simulink model "MotorImplementation"  (R2022a)
settings: Solver=FixedStepAuto  StartTime=0.0  StopTime=60  FixedStep=1/25  RelTol=1e-3
model workspace (MATLAB code in the model file):
  | %% Mechanical Parameters
  | d_Drum = 23.23e-2; % Meter
  | Drum_Friction = 0.001; % Ns/m
  | Drum_Inertia = 1.0; %kgm^2
  | 
  | n_sh = 5;
  | 
  | %% Load Case 1
  | Hs = 2.2; % m
  | T_w = 8.0; % s
  | m_payload = 8000; % kg
  | h_payload_0 = 75; % m
  | h_payload_final = h_payload_0; % m
  | h_seabed = 350; % m
  | 
  | %% Load Case 2
  | Hs = 2.2; % m
  | T_w = 8.0; % s
  | m_payload = 8000; % kg
  | h_payload_0 = 75; % m
  | h_payload_final = 15; % m
  | h_seabed = 350; % m
  | 
  | %% Load Case 3
  | Hs = 2.2; % m
  | T_w = 8.0; % s
  | m_payload = 8000; % kg
  | h_payload_0 =15; % m
  | h_payload_final = 0; % m
  | h_seabed = 350; % m
  | 
  | %% Sensors
  | % Noise simulation
  | sigma_w = 0.5; %m/s^2 (Standard deviation of noise)
  | beta = 10000; % Positive constant [-]
  | 
  | %% Payload parameters
  | % mass already defined (8000kg)
  | Volume_pl = 2; %m^3
  | Area_pl = 1.5; %m^2
  | C_D = 1.8; %[-] Drag coefficient
  | 
  | %syms rho vel
  | %F_drag = 0.5 * rho * vel^2 * C_D * Area_pl; % Density of sea water(surface) approx 1.025 kg/m^3, velocity comes from the simulation.
  | 
  | %% Seabed
  | k_spring = 1.8e6; %N/m
  | b_damper = 6.5e5; %Ns/m
  | rho = 1.025;
  | %syms delta_x
  | %if delta_x < 0
  | %    F_sb = 0;
  | %else
  | %    F_sb = k_spring*delta_x + b_damper*vel*sqrt(delta_x);
  | %end
  | 
  | %% Bouyant force
  | % The force pushing upwards when something floats down in water. Dependend
  | % on the fluid density, volume of the object falling and gravity
  | g = 9.81;
  | %F_boy = rho * Volume_pl * g;
  | 
  | %% Mechanical Parameters
  | T_N = 579 % Nominal torque [Nm]
  | PF_N = 0.85; % Nominal power factor
  | f=50;
  | n_N = 1483; % mechanical speed [rpm]
  | P_N = 90000 % Nominal mechanical power [W]
  | U = 400; % line-to-line rms stator voltage [V]
  | eta_N = 0.947; % efficiency
  | n_p = 2; % pole pairs
  | I_N=160;
  | 
  | %% Electrical parameters
  | % T-circuit
  | Rs = 0.04264;
  | L_sl = 0.3172;
  | Lm = 5.3031;
  | L_rl = 0.3172;
  | R_R = 0.0288;
  | psi_R = 20*P_N/(sqrt(2)*pi*n_p*I_N*n_N);
  | %Inv Gamma Transform
  | Lr = 5.3031 + 0.3172;
  | L_M = 5.3031^2/Lr;
  | L_M_hat = 5;
  | 
  | PSI_R = 5.3031/Lr * psi_R;
  | L_sigma =((5.3031+0.3172) - Lr);
  | %L_sigma_hat = 0.12;
  | RR = (5.3031/Lr)^2 * 0.0288;
  | %RR_Hat = 0.025;
  | R_R_opt = 0.0193;
  | X_M_opt = 2.81;
  | X_sig_opt = 0.0445;
  | 
  | R_R_hat = 0.02;
  | X_M_hat = 3;
  | X_sig_hat = 0.05;
  | R_s = 0.04264;
  | %% Control parameters
  | omega_bw = log(9)/1e-3;
  | kp = omega_bw * X_sig_hat;
  | ki = omega_bw^2 * X_sig_hat;
undefined symbols (not defined in the file): I_max, L_sigma_hat, magnitude, omega_1_N, psi_ref, R_hat, RR_Hat, Ts, V_base, w_BW
libraries: fl_lib x22, nesl_utility x10, CustomComponents_lib x6, slpidlib x4, simulink x3, eeTransforms x2, sdl_lib x1
(part 2 of 2)

== system MotorImplementation/Field Oriented Control/Velocity Controller ==
  omega_ref : Inport
  omega_rotor : Inport  Port=2
  PID Controller : slpidlib/PID Controller  Controller=PID  Form=Parallel  TimeDomain=Discrete-time  UseExternalTs=off  SampleTime=-1  IntegratorMethod=Forward Euler  FilterMethod=Forward Euler  ControllerParametersSource=internal  P=100  I=1000  UseKiTs=off  D=0  N=100  UseFilter=on  TunerSelectOption=Transfer Function Based (PID Tuner App)  InitialConditionSource=internal  InitialConditionForIntegrator=0  InitialConditionForFilter=0  DifferentiatorICPrevScaledInput=0  ExternalReset=none  TrackingMode=off  Kt=1  LimitOutput=off  SatLimitsSource=internal  UpperSaturationLimit=inf  LowerSaturationLimit=-inf  LinearizeAsGain=on  AntiWindupMode=none  Kb=1  POutMin=[]  POutMax=[]  IOutMin=[]  IOutMax=[]  DOutMin=[]  DOutMax=[]  NOutMin=[]  NOutMax=[]  SumOutMin=[]  SumOutMax=[]  SaturationOutMin=[]  SaturationOutMax=[]  PParamMin=[]  PParamMax=[]  IParamMin=[]  IParamMax=[]  DParamMin=[]  DParamMax=[]  NParamMin=[]  NParamMax=[]  KbParamMin=[]  KbParamMax=[]  KtParamMin=[]  KtParamMax=[]  KbOutMin=[]  KbOutMax=[]  KtOutMin=[]  KtOutMax=[]  IntegratorOutMin=[]  IntegratorOutMax=[]  FilterOutMin=[]  FilterOutMax=[]  SumI1OutMin=[]  SumI1OutMax=[]  SumI2OutMin=[]  SumI2OutMax=[]  SumI3OutMin=[]  SumI3OutMax=[]  SumI4OutMin=[]  SumI4OutMax=[]  SumDOutMin=[]  SumDOutMax=[]  DifferentiatorOutMin=[]  DifferentiatorOutMax=[]  FilterDiffOutCoefMin=[]  FilterDiffOutCoefMax=[]  ReciprocalOutMin=[]  ReciprocalOutMax=[]  SumDenOutMin=[]  SumDenOutMax=[]  SumNumOutMin=[]  SumNumOutMax=[]  DivideOutMin=[]  DivideOutMax=[]  UdiffTsProdOutMin=[]  UdiffTsProdOutMax=[]  NTsProdOutMin=[]  NTsProdOutMax=[]  UintegralTsProdOutMin=[]  UintegralTsProdOutMax=[]  UngainTsProdOutMin=[]  UngainTsProdOutMax=[]  IntegratorContinuousStateAttributes=''  IntegratorStateMustResolveToSignalObject=off  IntegratorRTWStateStorageClass=Auto  FilterContinuousStateAttributes=''  FilterStateMustResolveToSignalObject=off  FilterRTWStateStorageClass=Auto  ParallelPVariant=InternalParameters  IdealPVariant=Disabled  IVariant=InternalParameters  DVariant=InternalParameters  IntegratorVariant=Discrete  SatVariant=Disabled  AWVariant=Passthrough  PCopyVariant=Disabled  TRVariant=Disabled  FdbkBlocksVariant=Forward  IdealPFdbkVariant=Disabled  SatFdbkVariant=Disabled  DerivativeFilterVariant=ForwardEulerFilter  NVariant=InternalParameters  NCopyVariant=Disabled  FilterICVariant=InternalICsFilter  IntegratorICVariant=InternalICs  ExternalResetVariant=Disabled  TRSumVariant=Passthrough  SumFdbkVariant=Disabled  SumVariant=Sum_PID  TsampFilterVariant=InternalTs  TsampNgainVariant=Passthrough  TsampIntegralVariant=Passthrough  ExternalSaturationOutDataTypeStr=Inherit: Same as second input  aMode=0
  Scope : Scope  NumInputPorts=2
  Sum : Sum  Inputs=|+-
  iq_ref : Outport
  wires:
  omega_ref/1 -> Scope/1, Sum/1
  omega_rotor/1 -> Scope/2, Sum/2
  Sum/1 -> PID Controller/1
  PID Controller/1 -> iq_ref/1

== system MotorImplementation/Field Oriented Control/abc to dq ==
  i_a : Inport
  i_b : Inport  Port=2
  i_c : Inport  Port=3
  Rotor_electrical_angle : Inport  Port=4
  Park Transform : eeTransforms/Park Transform  AxisAlignment=Q-axis  PowerInvariant=off
  i_abc : Mux  Inputs=3
  i_dq : Outport
  wires:
  i_abc/1 -> Park Transform/1
  i_c/1 -> i_abc/3
  i_b/1 -> i_abc/2
  i_a/1 -> i_abc/1
  Rotor_electrical_angle/1 -> Park Transform/2
  Park Transform/1 -> i_dq/1

== system MotorImplementation/Field Oriented Control/dq to abc ==
  v_dq_sat : Inport
  Rotor_electrical_angle : Inport  Port=2
  Inverse Park Transform : eeTransforms/Inverse Park Transform  AxisAlignment=Q-axis  PowerInvariant=off
  V_abc : Outport
  wires:
  v_dq_sat/1 -> Inverse Park Transform/1
  Inverse Park Transform/1 -> V_abc/1
  Rotor_electrical_angle/1 -> Inverse Park Transform/2

== system MotorImplementation/FOC/IM-Model/Electromagnetic Torque ==
  i_s^s : Inport
  psi_R^s : Inport  Port=2
  conj : Math  Operator=conj
  T_em : Outport
  wires:
  psi_R^s/1 -> conj/1

== system MotorImplementation/FOC/IM-Model/Flux Equations ==
  psi_s^s : Inport
  psi_R^s : Inport  Port=2
  i_s^s : Outport
  i_R^s : Outport  Port=2

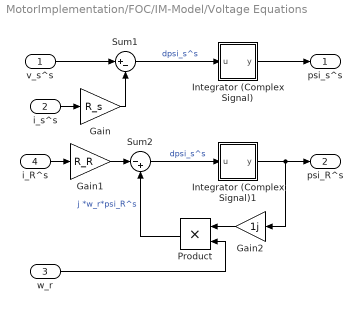
== system MotorImplementation/FOC/IM-Model/Voltage Equations ==
  v_s^s : Inport
  i_s^s : Inport  Port=2
  w_r : Inport  Port=3
  i_R^s : Inport  Port=4
  Gain : Gain  Gain=R_s
  Gain1 : Gain  Gain=R_R
  Gain2 : Gain  Gain=1j
  Integrator (Complex Signal) : Subsystem
      mask Display: disp('1/s');
  Integrator (Complex Signal)1 : Subsystem
      mask Display: disp('1/s');
  Product : Product  RndMeth=Zero
  Sum1 : Sum  Inputs=|+-
  Sum2 : Sum  Inputs=|-+
  psi_s^s : Outport
  psi_R^s : Outport  Port=2
  wires:
  w_r/1 -> Product/2
  Gain2/1 -> Product/1
  Integrator (Complex Signal)1/1(y) -> Gain2/1, psi_R^s/1
  Integrator (Complex Signal)/1(y) -> psi_s^s/1
  Gain/1 -> Sum1/2
  Sum1/1 -> Integrator (Complex Signal)/1(u)  "dpsi_s^s"
  i_s^s/1 -> Gain/1
  v_s^s/1 -> Sum1/1
  Product/1 -> Sum2/2  "j *w_r*psi_R^s"
  i_R^s/1 -> Gain1/1
  Gain1/1 -> Sum2/1
  Sum2/1 -> Integrator (Complex Signal)1/1(u)  "dpsi_s^s"

== system MotorImplementation/FOC/IM-Model/abc->alphabeta ==
  vs_abc : Inport
  Fcn : Fcn  Expr=2/3*(u(1)-0.5*u(2)-0.5*u(3))
  Fcn1 : Fcn  Expr=sqrt(3)/3*(u(2)-u(3))
  Real-Imag to Complex : RealImagToComplex
  v_s^s : Outport
  wires:
  Real-Imag to Complex/1 -> v_s^s/1
  Fcn1/1 -> Real-Imag to Complex/2  "beta"
  Fcn/1 -> Real-Imag to Complex/1  "alpha"
  vs_abc/1 -> Fcn/1, Fcn1/1

== system MotorImplementation/FOC/IM-Model/alphabeta->abc ==
  note: u(2)
  note: u(1)
  note: u(2)
  note: u(1)
  note: u(2)
  note: u(1)
  i_s^s : Inport
  Complex to Real-Imag : ComplexToRealImag
  Fcn : Fcn  Expr=u(1)
  Fcn1 : Fcn  Expr=-0.5*u(1)+0.5*sqrt(3)*u(2)
  Fcn2 : Fcn  Expr=-0.5*u(1)-0.5*sqrt(3)*u(2)
  Mux : Mux  Inputs=2
  Mux1 : Mux  Inputs=2
  Mux2 : Mux  Inputs=2
  Mux3 : Mux  Inputs=3
  is_abc : Outport
  wires:
  Mux3/1 -> is_abc/1
  Fcn2/1 -> Mux3/3
  Fcn1/1 -> Mux3/2
  Fcn/1 -> Mux3/1
  i_s^s/1 -> Complex to Real-Imag/1
  Mux2/1 -> Fcn2/1
  Mux1/1 -> Fcn1/1
  Complex to Real-Imag/2 -> Mux2/2, Mux1/2, Mux/2  "beta"
  Complex to Real-Imag/1 -> Mux2/1, Mux1/1, Mux/1  "alpha"
  Mux/1 -> Fcn/1

== system MotorImplementation/Field Oriented Control/Current Controller/PI Controller ==
  idq_ref : Inport
  i_dq : Inport  Port=2
  Complex to Real-Imag : ComplexToRealImag
  Gain : Gain  Gain=kp
  Gain1 : Gain  Gain=ki
  Integrator : Integrator
  Integrator1 : Integrator
  Real-Imag to Complex : RealImagToComplex
  Sum : Sum  Inputs=|++
  Sum1 : Sum  Inputs=|+-
  Controller Out : Outport
  wires:
  Complex to Real-Imag/1 -> Integrator/1
  Complex to Real-Imag/2 -> Integrator1/1
  Integrator/1 -> Real-Imag to Complex/1
  Integrator1/1 -> Real-Imag to Complex/2
  Real-Imag to Complex/1 -> Gain1/1
  Gain/1 -> Sum/1
  Gain1/1 -> Sum/2
  Sum/1 -> Controller Out/1
  idq_ref/1 -> Sum1/1
  i_dq/1 -> Sum1/2
  Sum1/1 -> Complex to Real-Imag/1, Gain/1

== system MotorImplementation/Field Oriented Control/IM/Flux Equation ==
  psi_s^s : Inport
  psi_R^s : Inport  Port=2
  Constant : Constant  Value=X_M_opt
  Eq(16) : Gain  Gain=1/X_sig_opt
  Eq(17) : Product  Inputs=*/
  Gain1 : Gain  Gain=X_M_opt/X_sig_opt
  Subtract : Sum  Inputs=+-
  Sum : Sum  Inputs=|+-
  i_s^s : Outport
  i_R^s : Outport  Port=2
  I_M : Outport  Port=3
  wires:
  psi_s^s/1 -> Eq(16)/1
  Eq(16)/1 -> Sum/1
  Sum/1 -> Subtract/2, i_s^s/1  "i_R = I_M^s - i_s^s"
  psi_R^s/1 -> Eq(17)/1
  Constant/1 -> Eq(17)/2
  Eq(17)/1 -> I_M/1, Subtract/1, Gain1/1  "I_M^s"
  Gain1/1 -> Sum/2
  Subtract/1 -> i_R^s/1

== system MotorImplementation/Field Oriented Control/IM/Torque_em ==
  psi_R^s : Inport
  i_s^s : Inport  Port=2
  Complex to Real-Imag1 : ComplexToRealImag
  Conjugate : Math  Operator=conj  SignedPower=on  RndMeth=Zero
  Gain : Gain  Gain=3*n_p/2
  Product : Product
  T_EM : Outport
  wires:
  i_s^s/1 -> Conjugate/1
  psi_R^s/1 -> Product/1
  Conjugate/1 -> Product/2
  Product/1 -> Complex to Real-Imag1/1
  Complex to Real-Imag1/2 -> Gain/1
  Gain/1 -> T_EM/1

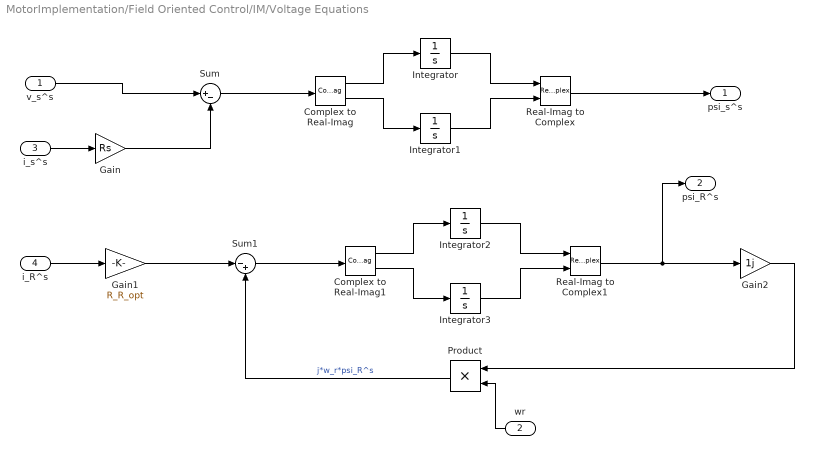
== system MotorImplementation/Field Oriented Control/IM/Voltage Equations ==
  v_s^s : Inport
  wr : Inport  Port=2
  i_s^s : Inport  Port=3
  i_R^s : Inport  Port=4
  Complex to Real-Imag : ComplexToRealImag
  Complex to Real-Imag1 : ComplexToRealImag
  Gain : Gain  Gain=Rs
  Gain1 : Gain  Gain=R_R_opt
  Gain2 : Gain  Gain=1j
  Integrator{,1..3} (4 alike) : Integrator
  Product : Product
  Real-Imag to Complex : RealImagToComplex
  Real-Imag to Complex1 : RealImagToComplex
  Sum : Sum  Inputs=|+-
  Sum1 : Sum  Inputs=|-+
  psi_s^s : Outport
  psi_R^s : Outport  Port=2
  wires:
  v_s^s/1 -> Sum/1
  i_s^s/1 -> Gain/1
  Gain/1 -> Sum/2
  Sum/1 -> Complex to Real-Imag/1
  Complex to Real-Imag/1 -> Integrator/1
  Complex to Real-Imag/2 -> Integrator1/1
  Integrator/1 -> Real-Imag to Complex/1
  Integrator1/1 -> Real-Imag to Complex/2
  Real-Imag to Complex/1 -> psi_s^s/1
  i_R^s/1 -> Gain1/1
  Gain1/1 -> Sum1/1
  Complex to Real-Imag1/2 -> Integrator3/1
  Integrator2/1 -> Real-Imag to Complex1/1
  Integrator3/1 -> Real-Imag to Complex1/2
  Real-Imag to Complex1/1 -> psi_R^s/1, Gain2/1
  Complex to Real-Imag1/1 -> Integrator2/1
  Sum1/1 -> Complex to Real-Imag1/1
  wr/1 -> Product/2
  Gain2/1 -> Product/1
  Product/1 -> Sum1/2  "j*w_r*psi_R^s"

== system MotorImplementation/FOC/IM-Model/Voltage Equations/Integrator (Complex Signal) ==
  u : Inport
  Complex to Real-Imag : ComplexToRealImag
  Integrator : Integrator  InitialCondition=psi_R
  Integrator1 : Integrator
  Real-Imag to Complex : RealImagToComplex
  y : Outport
  wires:
  u/1 -> Complex to Real-Imag/1
  Real-Imag to Complex/1 -> y/1
  Integrator1/1 -> Real-Imag to Complex/2
  Integrator/1 -> Real-Imag to Complex/1
  Complex to Real-Imag/2 -> Integrator1/1
  Complex to Real-Imag/1 -> Integrator/1

== system MotorImplementation/FOC/IM-Model/Voltage Equations/Integrator (Complex Signal)1 ==
  u : Inport
  Complex to Real-Imag : ComplexToRealImag
  Integrator : Integrator  InitialCondition=psi_R
  Integrator1 : Integrator
  Real-Imag to Complex : RealImagToComplex
  y : Outport
  wires:
  u/1 -> Complex to Real-Imag/1
  Real-Imag to Complex/1 -> y/1
  Integrator1/1 -> Real-Imag to Complex/2
  Integrator/1 -> Real-Imag to Complex/1
  Complex to Real-Imag/2 -> Integrator1/1
  Complex to Real-Imag/1 -> Integrator/1

== matlab function MotorImplementation/FOC/abc->dq1/MATLAB Function ==
  data: is_abc input size=3; thetas input size=1; is output size=2
function is = abc_dq(is_abc, thetas)
%#codegen

% Phase currents
ia = is_abc(1); ib = is_abc(2); ic = is_abc(3); 
is_abc = [ia;ib;ic];
% Space-vector transformation and coordinate transformation
T_dq = [cos(thetas), sin(thetas); -sin(thetas), cos(thetas)];
T_32 = [2/3, -1/3, -1/3; 0, 1/sqrt(3), -1/sqrt(3)];
is = T_dq*T_32*is_abc;   % Complete this

== matlab function MotorImplementation/Field Oriented Control/Current Controller/MATLAB Function ==
  data: i_q input; V_ph_max output; i_d input; omega_1 input
function V_ph_max = fcn(i_q, i_d, omega_1)

V_ph_max = abs(omega_1)*X_sig_opt*sqrt((i_q)^2 + ((X_sig_opt + X_M_opt)/X_sig_opt)^2 * i_d^2);

== matlab function MotorImplementation/DrawWork/Wave_Velocity/MATLAB Function ==
  settings: updateMethod=DISCRETE
  data: Hs input; T input; sim_time input; wave output; wave1 output
function [wave, wave1]  = fcn(Hs, T, sim_time)
%WAVE GEN generates stochastic waves
% Hs is the significant wave height [m]
% T is the mean period [s]
% t end is the end time [s]
% t is the time [s]
% wave is sea surface elevation [m]
%% Input parameters
w = linspace (0.1, 2.0, 20); % frequency range
delta_w = w(2) - w(1);
%% PM spectrum (freq. domain )
w1 = (2*pi)/T;
A = 0.11*(Hs^2)*(w1^4);
B = 0.44*(w1^4);
S = (A./w.^5).* exp(-(B./w.^4));
%% Wave amplitude (time domain)
%sfr = 1/25 ; % sampling frequency (Hz) (higher freq −> higher resolution)
t = sim_time; % time vector
phi_test = rng;
phi = 2*pi*(rand(1,length (w))-0.5); % random phase of ith frequency [rad]
rng(phi_test);
A_wave = sqrt(2*S.*delta_w); % amplitude of each sine wave. wave = [] ;

wave1 = [sum(A_wave .*cos(w.*t + phi))];
wave = [sum(A_wave .*-sin(w.*t + phi))];% [m] sea surface elevation  /Derivative

== matlab function MotorImplementation/DrawWork/Subsystem/MATLAB Function ==
  data: v input; F_D output
function F_D = fcn(v)
rho = 1.025;
C_D = 1.8;
Area_pl = 1.5; 


F_D =sign(v) * -(0.5*rho*v^2*C_D*Area_pl);

== matlab function MotorImplementation/Load Cases from matlab/Case Selector ==
  data: Case1 input; Case2 input; Case3 input; CaseSelector input; payload_ref_pos output
function payload_ref_pos  = fcn(Case1, Case2, Case3, CaseSelector)

if CaseSelector == 1
    payload_ref_pos = Case1;
    %select = "Case 1 in progress";
elseif CaseSelector == 2
    payload_ref_pos = Case2;
    %select = "Case 2 in progress";
elseif CaseSelector == 3
    payload_ref_pos = Case3;
    %select = "Case 3 in progress"; 
else 
    payload_ref_pos = 0;
    %select = "No Case is selected";  
end

== matlab function MotorImplementation/FOC/Current Controller/MATLAB Function ==
  data: v_sat_dq input size=2; i_s_ref input size=2; i_s input size=2; w_1 input size=1; I input size=1; w_BW parameter size=1; v_s_ref output size=2; Inew output; R_hat parameter size=1; L_sigma_hat parameter size=1; Ts parameter
function [v_s_ref, Inew] = cc(v_sat_dq,i_s_ref, i_s, w_1, I, w_BW, R_hat, L_sigma_hat, Ts)
%#codegen

%% Current controller 
% Gains
kp = 0; % Complete
ki = 0; % Complete
Ra = 0; % Complete

% Voltage reference in synchronous coordinates
i_s = i_s(1)+ 1i*i_s(2);
i_s_ref = i_s_ref(1)+ 1i*i_s_ref(2);
e = i_s_ref - i_s;
v_s_ref_c = 0; % complete: PI + active resistance Ra + decoupler.
v_s_ref = [real(v_s_ref_c);imag(v_s_ref_c)];

%% Update the integral state of the current controller 
v_sat_dq_c = v_sat_dq(1)+ 1i*v_sat_dq(2);
Inew = I + Ts*(e + (v_sat_dq_c)/kp);

== matlab function MotorImplementation/Control System ChouxWay/Current Controller/MATLAB Function ==
  data: v_sat_dq input size=2; i_s_ref input size=2; i_s input size=2; w_1 input size=1; I input size=1; w_BW parameter size=1; v_s_ref output size=2; Inew output; R_hat parameter size=1; L_sigma_hat parameter size=1; Ts parameter
function [v_s_ref, Inew] = cc(v_sat_dq,i_s_ref, i_s, w_1, I, w_BW, R_hat, L_sigma_hat, Ts)
%#codegen

%% Current controller 
% Gains
kp = 0; % Complete
ki = 0; % Complete
Ra = 0; % Complete

% Voltage reference in synchronous coordinates
i_s = i_s(1)+ 1i*i_s(2);
i_s_ref = i_s_ref(1)+ 1i*i_s_ref(2);
e = i_s_ref - i_s;
v_s_ref_c = 0; % complete: PI + active resistance Ra + decoupler.
v_s_ref = [real(v_s_ref_c);imag(v_s_ref_c)];

%% Update the integral state of the current controller 
v_sat_dq_c = v_sat_dq(1)+ 1i*v_sat_dq(2);
Inew = I + Ts*(e + (v_sat_dq_c)/kp);

== matlab function MotorImplementation/FOC/dq->abc/MATLAB Function ==
  data: vs_dq input size=2; thetas input size=1; vs_abc output size=3
function vs_abc = dq_abc(vs_dq, thetas)
%#codegen

% voltage in synchronous coordinates:
 vd = vs_dq(1); vq = vs_dq(2); 
vs_dq = [vd;vq];

% coordinate transformation and Space-vector transformation 
T_alphabeta = [cos(thetas), -sin(thetas); sin(thetas), cos(thetas)];
T_23 = [1, 0; -1/2, sqrt(3)/2; -1/2, -sqrt(3)/2];
vs_abc = T_23*T_alphabeta*vs_dq;   % Complete this
